simulink model "bolamagnetica"  (R2018a)
settings: Solver=VariableStepAuto  StartTime=0.0  StopTime=0.02  RelTol=1e-3
InitFcn:
  | m=0.5;
  | g=9.8;
  | R=2;
  | L=0.04;
  | K=8;
settings Model: Creator=ttorea  LastModifiedBy=ttorea

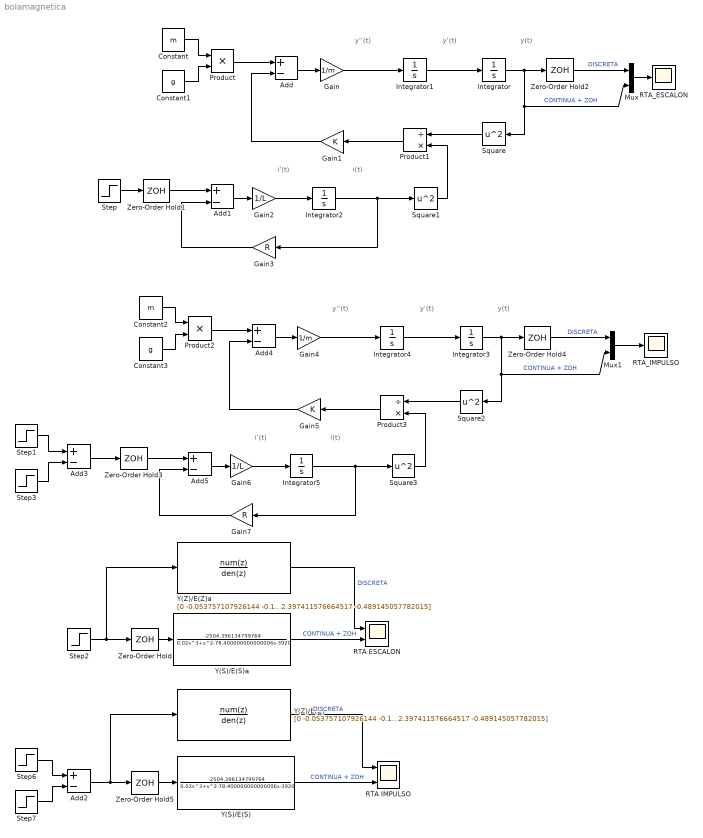
== system bolamagnetica ==
  note: i'(t)
  note: y(t)
  note: y'(t)
  note: y''(t)
  note: i(t)
  note: i(t)
  note: y(t)
  note: y'(t)
  note: y''(t)
  note: i'(t)
  Add{,1..5} (6 alike) : Sum  Inputs=+-
  Constant : Constant  Value=m
  Constant1 : Constant  Value=g
  Constant2 : Constant  Value=m
  Constant3 : Constant  Value=g
  Gain : Gain  Gain=1/m
  Gain1 : Gain  Gain=K
  Gain2 : Gain  Gain=1/L
  Gain3 : Gain  Gain=R
  Gain4 : Gain  Gain=1/m
  Gain5 : Gain  Gain=K
  Gain6 : Gain  Gain=1/L
  Gain7 : Gain  Gain=R
  Integrator : Integrator  InitialCondition=0.005
  Integrator{1..2,4..5} (4 alike) : Integrator
  Integrator3 : Integrator  InitialCondition=0.005
  Mux : Mux  Inputs=2
  Mux1 : Mux  Inputs=2
  Product : Product
  Product1 : Product  Inputs=/*
  Product2 : Product
  Product3 : Product  Inputs=/*
  RTA ESCALON : Scope  NumInputPorts=2
  RTA IMPULSO : Scope  NumInputPorts=2
  RTA_ESCALON : Scope
  RTA_IMPULSO : Scope
  Square{,1..3} (4 alike) : Math  Operator=square  SaturateOnIntegerOverflow=on
  Step : Step  Time=0  After=0.1106  SampleTime=0
  Step1 : Step  Time=0  After=2  SampleTime=0
  Step2 : Step  Time=0  After=2  SampleTime=0
  Step3 : Step  Time=0.00001  After=2  SampleTime=0
  Step6 : Step  Time=0  After=2  SampleTime=0
  Step7 : Step  Time=0.00001  After=2  SampleTime=0
  Y(S)/E(S) : TransferFcn  Numerator=[-2504.396134799764]  Denominator=[0.02 1 -78.400000000000006 -3920]
  Y(S)/E(S)a : TransferFcn  Numerator=[-2504.396134799764]  Denominator=[0.02 1 -78.400000000000006 -3920]
  Y(Z)/E(Z) : DiscreteTransferFcn  Numerator=[0 -0.053757107926144 -0.188445613408471 -0.037448542682446]  Denominator=[1 -3.345989984317626 2.397411576664517 -0.489145057782015]  SampleTime=0.0143
  Y(Z)/E(Z)a : DiscreteTransferFcn  Numerator=[0 -0.053757107926144 -0.188445613408471 -0.037448542682446]  Denominator=[1 -3.345989984317626 2.397411576664517 -0.489145057782015]  SampleTime=0.0143
  Zero-Order Hold{,1..5} (6 alike) : ZeroOrderHold  SampleTime=0.0143
  wires:
  Integrator1/1 -> Integrator/1
  Integrator/1 -> Zero-Order Hold2/1, Mux/2, Square/1  "CONTINUA + ZOH"
  Gain/1 -> Integrator1/1
  Add/1 -> Gain/1
  Constant/1 -> Product/1
  Constant1/1 -> Product/2
  Product/1 -> Add/1
  Gain1/1 -> Add/2
  Product1/1 -> Gain1/1
  Integrator2/1 -> Gain3/1, Square1/1
  Square1/1 -> Product1/2
  Gain2/1 -> Integrator2/1
  Add1/1 -> Gain2/1
  Gain3/1 -> Add1/2
  Square/1 -> Product1/1
  Zero-Order Hold/1 -> Y(S)/E(S)a/1
  Step2/1 -> Y(Z)/E(Z)a/1, Zero-Order Hold/1
  Zero-Order Hold1/1 -> Add1/1
  Zero-Order Hold2/1 -> Mux/1  "DISCRETA"
  Mux/1 -> RTA_ESCALON/1
  Y(S)/E(S)a/1 -> RTA ESCALON/2  "CONTINUA + ZOH"
  Y(Z)/E(Z)a/1 -> RTA ESCALON/1  "DISCRETA"
  Step6/1 -> Add2/1
  Step7/1 -> Add2/2
  Y(Z)/E(Z)/1 -> RTA IMPULSO/1  "DISCRETA"
  Zero-Order Hold5/1 -> Y(S)/E(S)/1
  Add2/1 -> Y(Z)/E(Z)/1, Zero-Order Hold5/1
  Y(S)/E(S)/1 -> RTA IMPULSO/2  "CONTINUA + ZOH"
  Step3/1 -> Add3/2
  Step1/1 -> Add3/1
  Step/1 -> Zero-Order Hold1/1
  Integrator4/1 -> Integrator3/1
  Mux1/1 -> RTA_IMPULSO/1
  Constant2/1 -> Product2/1
  Zero-Order Hold3/1 -> Add5/1
  Integrator3/1 -> Zero-Order Hold4/1, Mux1/2, Square2/1  "CONTINUA + ZOH"
  Square2/1 -> Product3/1
  Constant3/1 -> Product2/2
  Square3/1 -> Product3/2
  Add5/1 -> Gain6/1
  Gain5/1 -> Add4/2
  Zero-Order Hold4/1 -> Mux1/1  "DISCRETA"
  Gain4/1 -> Integrator4/1
  Add4/1 -> Gain4/1
  Gain7/1 -> Add5/2
  Product2/1 -> Add4/1
  Product3/1 -> Gain5/1
  Integrator5/1 -> Gain7/1, Square3/1
  Gain6/1 -> Integrator5/1
  Add3/1 -> Zero-Order Hold3/1
